simulink model "test"  (R2020a)
settings: Solver=VariableStepAuto  StartTime=0.0  StopTime=200  RelTol=1e-3
libraries: dspsrcs4 x1
settings Model: Creator=mike.don  LastModifiedBy=mike.don

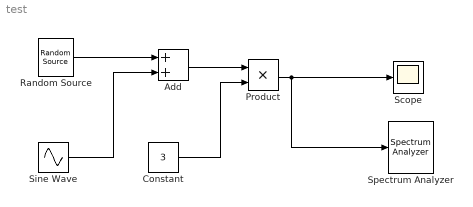
== system test ==
  Add : Sum
  Constant : Constant  Value=3
  Product : Product
  Random Source : dspsrcs4/Random Source  SrcType=Gaussian  NormMethod=Ziggurat  CltLength=12  MinVal=0  MaxVal=1  MeanVal=0  VarVal=0.2  RepMode=Not repeatable  rawSeed=1  IsInherit=off  SampMode=Discrete  SampTime=0.1  SampFrame=1  DataType=Double  OutComplex=Real  OutputFrames=off
  Scope : Scope
  Sine Wave : Sin  Frequency=0.5  SampleTime=0.2
  Spectrum Analyzer : SpectrumAnalyzer
  wires:
  Random Source/1 -> Add/1
  Add/1 -> Product/1
  Sine Wave/1 -> Add/2
  Constant/1 -> Product/2
  Product/1 -> Spectrum Analyzer/1, Scope/1
